simulink model "msk"  (Simulink 5.0)
settings: Solver=ode45  StartTime=0.0  StopTime=0.05  RelTol=1e-3
libraries: dspsigops x4, dspbuff3 x2, dspsigattribs x2, simulink x1, commrandsrc2 x1
settings Model: LastModifiedBy=Daiming Qu

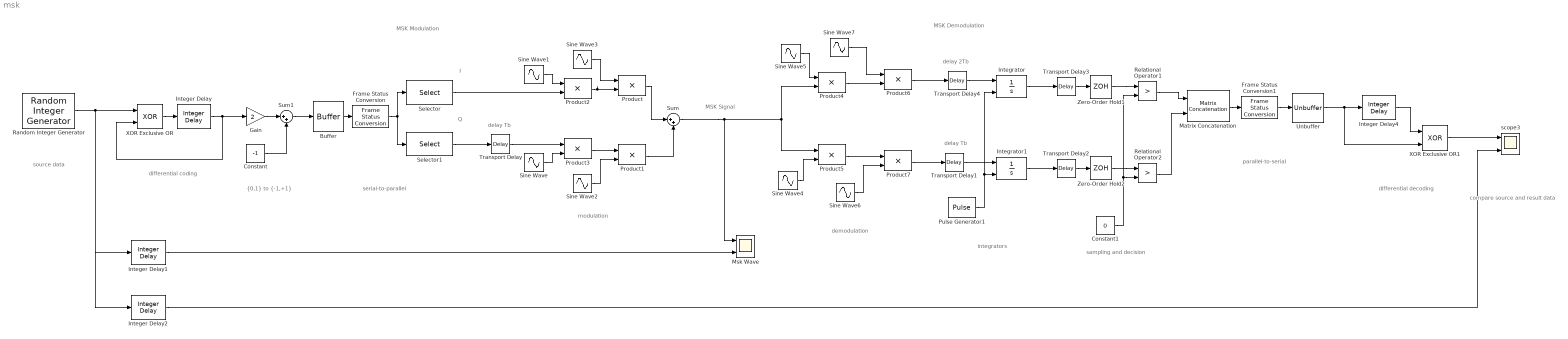
== system msk ==
  note: MSK Signal
  note: MSK Modulation
  note: serial-to-parallel
  note: delay Tb
  note: {0,1} to {-1,+1}
  note: differential coding
  note: modulation
  note: demodulation
  note: delay 2Tb
  note: integrators
  note: delay Tb
  note: MSK Demodulation
  note: sampling and decision
  note: parallel-to-serial
  note: differential decoding
  note: source data
  note: compare
      | source
      | and
      | result
      | data
  note: I
  note: Q
  Buffer : dspbuff3/Buffer  N=2  V=0  ic=0
  Constant : Constant  Value=-1
  Constant1 : Constant  Value=0
  Frame Status Conversion : dspsigattribs/Frame Status Conversion  growRefPort=off  outframe=Sample-based
  Frame Status Conversion1 : dspsigattribs/Frame Status Conversion  growRefPort=off  outframe=Frame-based
  Gain : Gain  Gain=2  SaturateOnIntegerOverflow=on
  Integer Delay : dspsigops/Integer Delay  delay=1  ic=0  reset_popup=None
  Integer Delay1 : dspsigops/Integer Delay  delay=3  ic=0  reset_popup=None
  Integer Delay2 : dspsigops/Integer Delay  delay=7  ic=0  reset_popup=None
  Integer Delay4 : dspsigops/Integer Delay  delay=1  ic=0  reset_popup=None
  Integrator : Integrator  ExternalReset=rising
  Integrator1 : Integrator  ExternalReset=rising
  Matrix Concatenation : simulink/Math Operations/Matrix Concatenation  numInports=2  catMethod=Vertical
  Msk Wave : Scope  NumInputPorts=2
      settings: YMin=-5~-2  YMax=5~2
  Product{,1..7} (8 alike) : Product  SaturateOnIntegerOverflow=on
  Pulse Generator1 : DiscretePulseGenerator  PulseType=Time based  Period=0.002  PulseWidth=50
  Random Integer Generator : commrandsrc2/Random Integer Generator  mul=2  seed=37  Ts=1/1000  frameBased=off  sampPerFrame=1  orient=off
  Relational Operator1 : RelationalOperator  Operator=>  ShowAdditionalParam=on
  Relational Operator2 : RelationalOperator  Operator=>  ShowAdditionalParam=on
  Selector : Selector  InputType=Matrix  Elements=[1]  InputPortWidth=2
  Selector1 : Selector  InputType=Matrix  Elements=[2]  Rows=2  InputPortWidth=2
  Sine Wave : Sin  Frequency=pi/2*1000  Phase=-3/2*pi  SampleTime=1/100000
  Sine Wave1 : Sin  Frequency=pi/2*1000  Phase=-3/2*pi+pi/2  SampleTime=1/100000
  Sine Wave2 : Sin  Frequency=1000*2*pi  SampleTime=1/100000
  Sine Wave3 : Sin  Frequency=1000*2*pi  Phase=pi/2  SampleTime=1/100000
  Sine Wave4 : Sin  Frequency=1000*2*pi  SampleTime=1/100000
  Sine Wave5 : Sin  Frequency=1000*2*pi  Phase=pi/2  SampleTime=1/100000
  Sine Wave6 : Sin  Frequency=pi/2*1000  Phase=-3/2*pi  SampleTime=1/100000
  Sine Wave7 : Sin  Frequency=pi/2*1000  Phase=-3/2*pi+pi/2  SampleTime=1/100000
  Sum : Sum  Inputs=|++  SaturateOnIntegerOverflow=on
  Sum1 : Sum  Inputs=|++  SaturateOnIntegerOverflow=on
  Transport Delay : TransportDelay  DelayTime=0.001  BufferSize=10
  Transport Delay1 : TransportDelay  DelayTime=0.001001  BufferSize=10
  Transport Delay2 : TransportDelay  DelayTime=0.00000001  BufferSize=10
  Transport Delay3 : TransportDelay  DelayTime=0.00000001  BufferSize=10
  Transport Delay4 : TransportDelay  DelayTime=0.002  BufferSize=10
  Unbuffer : dspbuff3/Unbuffer  ic=0
  XOR Exclusive OR : Logic  Operator=XOR  ShowAdditionalParam=on  AllPortsSameDT=off  OutDataTypeMode=Specify via dialog
  XOR Exclusive OR1 : Logic  Operator=XOR  ShowAdditionalParam=on  AllPortsSameDT=off  OutDataTypeMode=Specify via dialog
  Zero-Order Hold1 : ZeroOrderHold  SampleTime=0.002
  Zero-Order Hold2 : ZeroOrderHold  SampleTime=0.002
  scope3 : Scope  NumInputPorts=2
      settings: YMin=-5~-5  YMax=5~5
  wires:
  Product2/1 -> Product/2
  Product3/1 -> Product1/1
  Transport Delay/1 -> Product3/1
  Sum/1 -> Product5/1, Product4/2, Msk Wave/1
  Integrator/1 -> Transport Delay3/1
  Integrator1/1 -> Transport Delay2/1
  XOR Exclusive OR1/1 -> scope3/1
  Integer Delay2/1 -> scope3/2
  Integer Delay1/1 -> Msk Wave/2
  XOR Exclusive OR/1 -> Integer Delay/1
  Gain/1 -> Sum1/1
  Sine Wave/1 -> Product3/2
  Sine Wave3/1 -> Product/1
  Sine Wave2/1 -> Product1/2
  Product4/1 -> Product6/2
  Product5/1 -> Product7/1
  Sine Wave4/1 -> Product5/2
  Sine Wave5/1 -> Product4/1
  Sine Wave7/1 -> Product6/1
  Sine Wave6/1 -> Product7/2
  Pulse Generator1/1 -> Integrator/2, Integrator1/2
  Zero-Order Hold2/1 -> Relational Operator2/1
  Zero-Order Hold1/1 -> Relational Operator1/1
  Integer Delay4/1 -> XOR Exclusive OR1/1
  Random Integer Generator/1 -> Integer Delay1/1, Integer Delay2/1, XOR Exclusive OR/1
  Integer Delay/1 -> XOR Exclusive OR/2, Gain/1
  Sum1/1 -> Buffer/1
  Selector1/1 -> Transport Delay/1
  Buffer/1 -> Frame Status Conversion/1
  Frame Status Conversion/1 -> Selector/1, Selector1/1
  Selector/1 -> Product2/2
  Product/1 -> Sum/1
  Product1/1 -> Sum/2
  Sine Wave1/1 -> Product2/1
  Product7/1 -> Transport Delay1/1
  Transport Delay1/1 -> Integrator1/1
  Product6/1 -> Transport Delay4/1
  Transport Delay4/1 -> Integrator/1
  Transport Delay2/1 -> Zero-Order Hold2/1
  Transport Delay3/1 -> Zero-Order Hold1/1
  Frame Status Conversion1/1 -> Unbuffer/1
  Matrix Concatenation/1 -> Frame Status Conversion1/1
  Relational Operator1/1 -> Matrix Concatenation/1
  Constant1/1 -> Relational Operator1/2, Relational Operator2/2
  Relational Operator2/1 -> Matrix Concatenation/2
  Unbuffer/1 -> Integer Delay4/1, XOR Exclusive OR1/2
  Constant/1 -> Sum1/2
